simulink library "INT_ACSwt_DD"  (R2016b)
settings: Solver=VariableStepAuto  StartTime=0.0  StopTime=10.0  RelTol=1e-3
settings Model: Creator=lenovo  LastModifiedBy=lenovo

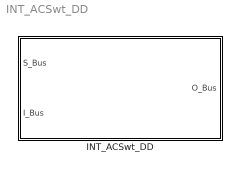
== system INT_ACSwt_DD ==
  INT_ACSwt_DD : Subsystem

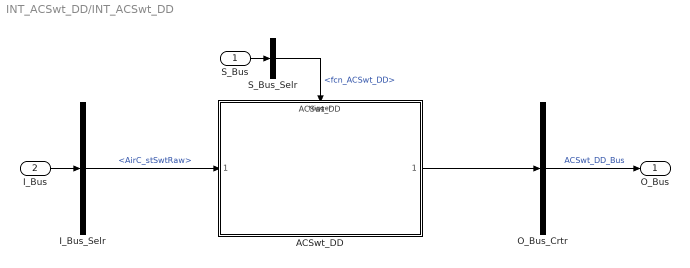
== system INT_ACSwt_DD/INT_ACSwt_DD ==
  S_Bus : Inport
  I_Bus : Inport  Port=2
  ACSwt_DD : ModelReference  ModelNameDialog=ACSwt_DD  SimulationMode=Normal  ModelReferenceVersion=1.11  TriggerPortName=function  TriggerPortTriggerType=function-call  TriggerPortStatesWhenEnabling=held
  I_Bus_Selr : BusSelector  OutputSignals=AirC_stSwtRaw
  O_Bus_Crtr : BusCreator  Inputs=1
  S_Bus_Selr : BusSelector  OutputSignals=fcn_ACSwt_DD
  O_Bus : Outport
  wires:
  S_Bus_Selr/1 -> ACSwt_DD/Trigger  "<fcn_ACSwt_DD>"
  S_Bus/1 -> S_Bus_Selr/1
  I_Bus/1 -> I_Bus_Selr/1
  I_Bus_Selr/1 -> ACSwt_DD/1  "<AirC_stSwtRaw>"
  O_Bus_Crtr/1 -> O_Bus/1  "ACSwt_DD_Bus"
  ACSwt_DD/1 -> O_Bus_Crtr/1
